simulink model "sim_1_filtering"  (R2021a)
settings: Solver=FixedStepDiscrete  StartTime=0.0  StopTime=inf  RelTol=1e-3
undefined symbols (not defined in the file): fdesignblkfcn, gcbh
libraries: dspsrcs4 x2, dspsigops x1, dspspect3 x1
settings Model: Creator=vpixx  LastModifiedBy=vpixx
settings SolverCC: AlgebraicLoopSolver=TrustRegion  AutoInsertRateTranBlk=on
settings DataIOCC: LimitDataPoints=on  SaveOutput=off  SignalLogging=off  SaveTime=off
settings OptimizationCC: LifeSpan=inf  SimCompilerOptimization=on
settings DebuggingCC: AlgebraicLoopMsg=error  SingleTaskRateTransMsg=error  AllowSymbolicDim=off  SFUnexpectedBacktrackingDiag=warning  SFNoUnconditionalDefaultTransitionDiag=warning  SFExecutionAtInitializationDiag=none  SFMachineParentedDataDiag=warning  ArithmeticOperatorsInVariantConditions=warning
settings SFSimCC: SimUseLocalCustomCode=off  CustomCodeUndefinedFunction=UseInterfaceOnly
settings RTWCC: RTWUseLocalCustomCode=off
settings CodeAppCC: StateflowObjectComments=on
settings GRTTargetCC: TargetLangStandard=C89/C90 (ANSI)
settings ConfigComp: CovMetricSettings=dw  CovSaveCumulativeToWorkspaceVar=on  CovSaveSingleToWorkspaceVar=on  CovExternalEMLEnable=off  CovSFcnEnable=off

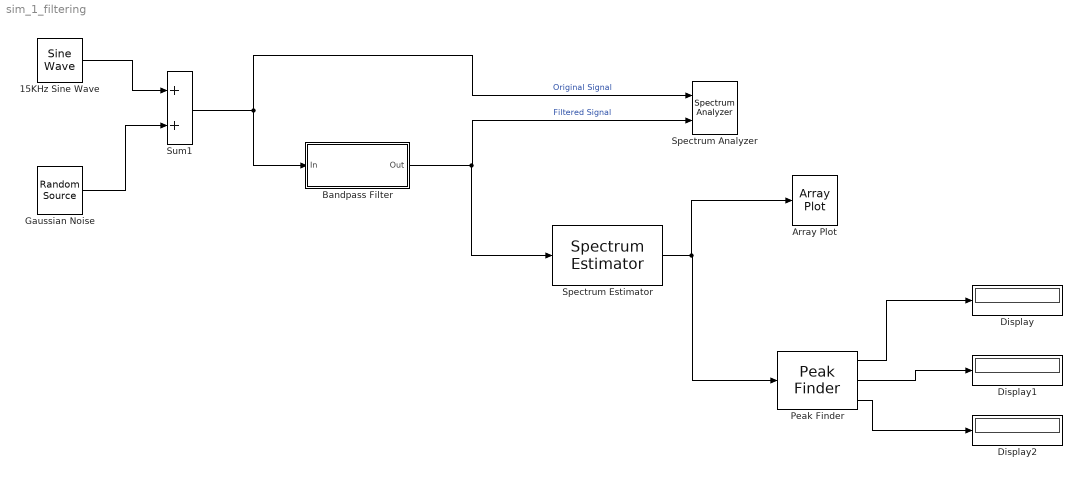
== system sim_1_filtering ==
  15KHz Sine Wave : dspsrcs4/Sine Wave  Amplitude=1  Frequency=15000  Phase=0  SampleMode=Discrete  OutComplex=Real  CompMethod=Trigonometric fcn  TableSize=Speed  SampleTime=1/44100  SamplesPerFrame=256  ResetState=Restart at time zero  OutputFrames=off  dataType=double  wordLen=16  udDataType=sfix(16)  fracBitsMode=Best precision  numFracBits=15  OutDataTypeStr=double  LastOutDataTypeStr=double
  Array Plot : ArrayPlot  WindowPosition=[-1253.000000,1244.000000,1078.000000,713.000000,]  Visible=on  YLimits=[-102.77974374870404,36.83955517089829]  DefaultConfigurationName=dsp.scopes.ArrayPlotBlockSpecification
  Bandpass Filter : Subsystem  DialogController=fdesignblkfcn  InitFcn=fdesignblkfcn(gcbh, {'InitFcn'});  mask(Bandpass Filter){}
      mask help: Design a bandpass filter
      settings: CopyFcn=fdesignblkfcn(gcbh, {'CopyFcn'});
      mask Help: helpview(mapfilelocation('dsp'), 'dspbandpassfilter');
      mask Display: disp('Bandpass');
  Display : Display
  Display1 : Display
  Display2 : Display
  Gaussian Noise : dspsrcs4/Random Source  SrcType=Gaussian  NormMethod=Ziggurat  CltLength=12  MinVal=0  MaxVal=1  MeanVal=0  VarVal=.05  RepMode=Specify seed  rawSeed=1234567  IsInherit=off  SampMode=Discrete  SampTime=1/44100  SampFrame=256  DataType=Double  OutComplex=Real  OutputFrames=off
  Peak Finder : dspsigops/Peak Finder  polarity=Maxima  indexBase=Zero  outputIdx=on  outputVal=on  maxPeaks=1  NoiseDistinguish=off  thresh=0  roundingMode=Floor  overflowMode=off
      settings: SourceProductBaseCode=DS  allowOverrides=off
  Spectrum Analyzer : SpectrumAnalyzer  NumInputPorts=2
  Spectrum Estimator : dspspect3/Spectrum Estimator  Method=Welch  NumTapsPerBand=12  SpectrumType=Power  FrequencyResolutionMethod=Auto  FilterBankResolutionMethod=Auto  RBW=5  WindowLength=1024  FrequencyBandsSource=Same as input frame size  FrequencyBands=1024  FFTLengthSource=Auto  FFTLength=1024  InheritSampleRate=on  SampleRate=44100  Window=Hann  SidelobeAttenuation=60  AveragingMethod=Running  SpectralAverages=10  ForgettingFactorPort=off  ForgettingFactor=0.9  Overlap=0  ReferenceLoad=1  FrequencyRange=Centered  PowerUnits=dBm  OutputMaxHoldSpectrum=off  OutputMinHoldSpectrum=off  OutputFrequencyVector=off  OutputRBW=off  SimulateUsing=Code generation
      settings: SourceProductBaseCode=DS
  Sum1 : Sum
  wires:
  Sum1/1 -> Spectrum Analyzer/1, Bandpass Filter/1(In)  "Original Signal"
  Bandpass Filter/1(Out) -> Spectrum Estimator/1, Spectrum Analyzer/2  "Filtered Signal"
  15KHz Sine Wave/1 -> Sum1/1
  Gaussian Noise/1 -> Sum1/2
  Peak Finder/2 -> Display1/1
  Peak Finder/3 -> Display2/1
  Peak Finder/1 -> Display/1
  Spectrum Estimator/1 -> Array Plot/1, Peak Finder/1

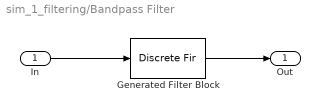
== system sim_1_filtering/Bandpass Filter ==
  In : Inport
  Generated Filter Block : DiscreteFir  Tag=BlockMethodSubSystem  Coefficients=[0.00030509485780131837 -0.000263792126378913625 -0.000172803533790532302 -0.000190040515952262593 9.66008454810429042e-06 -2.28686922643974567e-05 -0.000248137580884423732 0.000232486829361674182 1.90758230425352307e-05 -0.000467169326614204675 0.000536547169435503887 -3.20887604728390546e-06 -0.000788570967392656806 0.000965585829033094702 -9.96188840210191146e-05 -0.00117575175307841327 0.00152711595781212183 -0.000291615593583341773 -0.00158714796954679454 0.00220170139852316881 -0.000594836923800829624 -0.00197176055853910378 0.00294358027484212421 -0.00100873695079197281 -0.00227299495774071396 0.00368075011160656643 -0.00150896263248237309 -0.00243776790950764538 0.00432070894845473091 -0.00204320838728673732 -0.00242632161923963391 0.00475949270087260446 -0.00253131677056271697 -0.00222290146700881638 0.00489553314682639271 -0.00287141679252382164 -0.00184263848815814321 0.0046438795709538086 -0.00294870233910481203 -0.00133720874288083464 0.00395423057910180686 -0.00265391084853835004 -0.000790390224752670332 0.00282445668366836404 -0.00190245135088390623 -0.000309460978634241686 0.00130953443279841083 -0.000653476394312576354 -1.15235885088159268e-05 -0.00047610703037464857 0.00107103834955507332 6.69827109565989855e-07 -0.00236810133819034775 0.00317376357072063093 -0.000340878836527780556 -0.00416503257532557444 0.00548001342387485595 -0.00104724913974824823 -0.0056571462678133037 0.00774468800632957793 -0.00205415508311651085 -0.00665190932831504541 0.00967067818353547354 -0.00321631408638481777 -0.00700831771569008621 0.0109397005528373489 -0.00430817620251710935 -0.00666102302473576754 0.0112488059705813798 -0.00504245108313032195 -0.00564346525016347789 0.010350218492060477 -0.00509696326240598532 -0.0040923494422564809 0.00809165614012743832 -0.00415266553840342324 -0.00224358346615625677 0.00444523897357911122 -0.00193901622113542183 -0.000409666242419861031 -0.000473857968713486326 0.00172487656646395254 0.00105493563216371841 -0.00640429152399130119 0.00689156451316284922 0.00179740958745367167 -0.0129574531743384506 0.0134605198142113951 0.00151440516991980991 -0.0196493895971220668 0.0211702443269451007 -1.22595956362336961e-06 -0.025948341281038817 0.0296092769565176085 -0.00282569780805533646 -0.0313319425146961136 0.0382459513168980011 -0.00688195413152562288 -0.0353447734021454865 0.0464763796802021983 -0.0119361588443873522 -0.037649619902350967 0.05368284366609858 -0.0176153824373732337 -0.0380675618885435579 0.0592983046137666239 -0.0234425572346868387 -0.0365994784228061906 0.0628656689023892878 -0.0288876568007945429 -0.0334262637934190712 0.0640890734910454229 -0.0334262637934190712 -0.0288876568007945429 0.0628656689023892878 -0.0365994784228061906 -0.0234425572346868387 0.0592983046137666239 -0.0380675618885435579 -0.0176153824373732337 0.05368284366609858 -0.037649619902350967 -0.0119361588443873522 0.0464763796802021983 -0.0353447734021454865 -0.00688195413152562288 0.0382459513168980011 -0.0313319425146961136 -0.00282569780805533646 0.0296092769565176085 -0.025948341281038817 -1.22595956362336961e-06 0.0211702443269451007 -0.0196493895971220668 0.00151440516991980991 0.0134605198142113951 -0.0129574531743384506 0.00179740958745367167 0.00689156451316284922 -0.00640429152399130119 0.00105493563216371841 0.00172487656646395254 -0.000473857968713486326 -0.000409666242419861031 -0.00193901622113542183 0.00444523897357911122 -0.00224358346615625677 -0.00415266553840342324 0.00809165614012743832 -0.0040923494422564809 -0.00509696326240598532 0.010350218492060477 -0.00564346525016347789 -0.00504245108313032195 0.0112488059705813798 -0.00666102302473576754 -0.00430817620251710935 0.0109397005528373489 -0.00700831771569008621 -0.00321631408638481777 0.00967067818353547354 -0.00665190932831504541 -0.00205415508311651085 0.00774468800632957793 -0.0056571462678133037 -0.00104724913974824823 0.00548001342387485595 -0.00416503257532557444 -0.000340878836527780556 0.00317376357072063093 ...(+1273 chars)]  InputProcessing=Columns as channels (frame based)
  Out : Outport  VectorParamsAs1DForOutWhenUnconnected=off
  wires:
  In/1 -> Generated Filter Block/1
  Generated Filter Block/1 -> Out/1
